simulink library "lib6DOFUtilityEquations"  (R2020b)
settings: Solver=VariableStepAuto  StartTime=0.0  StopTime=10.0  RelTol=1e-3
undefined symbols (not defined in the file): Earth, outputs, WGS84
libraries: aerolibtransform2 x1
settings Model: Creator=caatay  LastModifiedBy=caatay

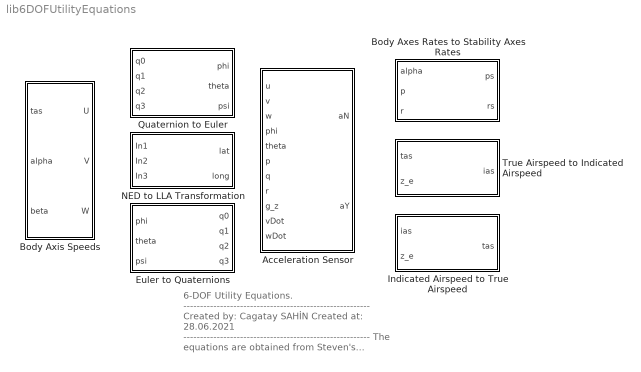
== system lib6DOFUtilityEquations ==
  note: 6-DOF Utility Equations.
      | --------------------------------------------------------
      | Created by: Cagatay SAHİN
      | Created at: 28.06.2021
      | --------------------------------------------------------
      | The equations are obtained from
      | Steven's textbook.
      | The reference book can be found in
      | "references folder".
      | --------------------------------------------------------
      | for question:
      | cagataysahin44@gmail.com
  Acceleration Sensor : Subsystem  mask(EOM Models - Utility Equations - Acceleration Sensor){}
      mask help: This block calculates acceleration information in SI Units.
      mask Help:
      | This block can calculate aircaft's acceleration data with using force and weight information
      | -------------------------------------------------------------------------------------------------------------------------------------------------
      | Inputs of this block:
      | 	u: X-Axis body speed (ft/sec)
      | 	v: Y-Axis body speed (ft/sec)
      | 	w: Z-Axis body speed (ft/sec)
      | 	phi: Roll Angle (rad)
      | 	theta: Pitch Angle (rad)
      | 	p: Body axis roll rate (ft/sec^2)
      | 	q: Body axis pitch rate (ft/sec^2)
      | 	r: Body axis yaw rate (ft/sec^2)
      | 	g_z: Z-Axis gravitional force (ft/sec^2)
      | 	vDot: Derivative of Y-Axis Body Speed (ft/sec^2)
      | 	wDot : Derivative of Z-Axis Body Speed (ft/sec^2)
      | Outputs of this block:
      | 	Aircraft acceleration: Z and Y acceleration [ft/sec^2].
      | -------------------------------------------------------------------------------------------------------------------------------------------------
      | Equations that in this block can be found in Steven's textbook. This textbook is in "literature" subfolder.
      | for question: "cagataysahin44@gmail.com".
      mask Display:
      | port_label('input',1,'u','texmode','on');
      | port_label('input',2,'v','texmode','on');
      | port_label('input',3,'w','texmode','on');
      | port_label('input',4,'\phi','texmode','on');
      | port_label('input',5,'\theta','texmode','on');
      | port_label('input',6,'p','texmode','on');
      | port_label('input',7,'q','texmode','on');
      | port_label('input',8,'r','texmode','on');
      | port_label('input',9,'g_{z}','texmode','on');
      | port_label('input',10,'v_{der}','texmode','on');
      | port_label('input',11,'w_{der}','texmode','on');
      | 
      | port_label('output',1,'a_{N}','texmode','on');
      | port_label('output',2,'a_{Y}','texmode','on');
  Body Axes Rates to Stability Axes Rates : Subsystem  mask(EOM Model - Utility Equations - Body Axes Rates to Stability Axes Rates){}
      mask help: Aircraft's stability axes angular rates calculation with using body axes angular rates and wind parameters alpha.
      mask Help:
      | This block can calculate aircaft's stability axes angular rates with using state information
      | -------------------------------------------------------------------------------------------------------------------------------------------------
      | Inputs of this block:
      | 	alpha: Angle of attack (rad).
      | 	p: Body axis roll rate (rad/s).
      | 	r: Body axis yaw rate (rad/s):
      | Outputs of this block:
      | 	p_s: Stability axis roll rate (rad/s).
      | 	r_s: Stabiltiy axis yaw rate (rad/s).
      | -------------------------------------------------------------------------------------------------------------------------------------------------
      | Equations that in this block can be found in Steven's textbook. This textbook is in "literature" subfolder.
      | for question: "cagataysahin44@gmail.com".
      mask Display:
      | port_label('input',1,'\alpha','texmode','on');
      | port_label('input',2,'p','texmode','on');
      | port_label('input',3,'r','texmode','on');
      | 
      | port_label('output',1,'p_{s}','texmode','on');
      | port_label('output',2,'r_{s}','texmode','on');
  Body Axis Speeds : Subsystem  mask(EOM Model - Utility Equations - Wind Paramaters to Body Axis Speeds.){}
      mask help: To Convert aircaft's wind parameters to body axis speeds which is coordinate transfer.
      mask Help:
      | This block can calculate aircaft's body axis speed which transforming wind axis coordinate to body axis coordinate.
      | -------------------------------------------------------------------------------------------------------------------------------------------------
      | Inputs of this block:
      | 	Wind Axis Params: Tas, AoA, AoS [ft/sec, rad].
      | Outputs of this block:
      | 	Body Axis Speeds: U, V, W body axis speeds [ft/sec].
      | -------------------------------------------------------------------------------------------------------------------------------------------------
      | Equations that in this block can be found in Steven's textbook. This textbook is in "literature" subfolder.
      | for question: "cagataysahin44@gmail.com".
      mask Display:
      | port_label('input',1,'V_{tas}','texmode','on');
      | port_label('input',2,'\alpha','texmode','on');
      | port_label('input',3,'\beta','texmode','on');
      | 
      | port_label('output',1,'U','texmode','on');
      | port_label('output',2,'V','texmode','on');
      | port_label('output',3,'W','texmode','on');
  Euler to Quaternions : Subsystem  mask(EOM Model - Utility Equations - Euler Angle to Quaternion Angle Transformation){}
      mask help: This function converts euler angles to quaternion angles.
      mask Help:
      | This block can transform euler angles to quaternion angles.
      | -------------------------------------------------------------------------------------------------------------------------------------------------
      | Inputs of this block:
      | 	Euler angles [rad].
      | Outputs of this block:
      | 	Quaternion angles [rad].
      | -------------------------------------------------------------------------------------------------------------------------------------------------
      | Equations that in this block can be found in Steven's textbook. This textbook is in "literature" subfolder.
      | for question: "cagataysahin44@gmail.com".
      mask Display:
      | port_label('input',1,'\phi','texmode','on');
      | port_label('input',2,'\theta','texmode','on');
      | port_label('input',3,'\psi','texmode','on');
      | 
      | port_label('output',1,'q_{0}','texmode','on');
      | port_label('output',2,'q_{1}','texmode','on');
      | port_label('output',3,'q_{2}','texmode','on');
      | port_label('output',4,'q_{3}','texmode','on');
  Indicated Airspeed to True Airspeed : Subsystem  mask(EOM Models - Utility Equations - IAS to TAS Conversion){}
      mask help: Aircraft's Lo-Fi True Airspeed calculation with using altitude and indicated airspeed information.
      mask Help:
      | This block can calculate aircaft's true airspeed with using state information.
      | -------------------------------------------------------------------------------------------------------------------------------------------------
      | Inputs of this block:
      | 	V_ias: Indicated airspeed (ft/sec)
      | 	z_e: Altitude (ft)
      | Outputs of this block:
      | 	V_tas: True airspeed (ft/sec)
      | -------------------------------------------------------------------------------------------------------------------------------------------------
      | Equations that in this block can be found in Steven's textbook. This textbook is in "literature" subfolder.
      | for question: "cagataysahin44@gmail.com".
      mask Display:
      | port_label('input',1,'V_{ias}','texmode','on');
      | port_label('input',2,'z_{e}','texmode','on');
      | 
      | port_label('output',1,'V_{tas}','texmode','on');
  NED to LLA Transformation : Subsystem  mask(EOM Model - Utility Equations -  NED tol LLA Transformation Model){}
      mask help: This function converts ned position variables (x,y,z) into lla (latitude, longitude, altitude) parameters.
      mask Help:
      | This block can transform North,East,Down values to Lattitude and Longitude angles.
      | -------------------------------------------------------------------------------------------------------------------------------------------------
      | Inputs of this block:
      | 	ned: North, East, Down values (ft).
      | Outputs of this block:
      | 	LLA: Latitude, Longitude (deg).
      | -------------------------------------------------------------------------------------------------------------------------------------------------
      | Equations that in this block can be found in Steven's textbook. This textbook is in "literature" subfolder.
      | for question: "cagataysahin44@gmail.com".
      mask Display:
      | port_label('input',1,'x_{e}','texmode','on');
      | port_label('input',2,'y_{e}','texmode','on');
      | port_label('input',3,'e_{e}','texmode','on');
      | 
      | port_label('output',1,'\mu','texmode','on');
      | port_label('output',2,'l','texmode','on');
  Quaternion to Euler : Subsystem  mask(EOM Model - Utility Equations -  Quaternion Angle to Euler Angle Transformation){}
      mask help: This function converts quaternion angles to euler angles.
      mask Help:
      | This block can transform quaternion angles to euler angles.
      | -------------------------------------------------------------------------------------------------------------------------------------------------
      | Inputs of this block:
      | 	Quaternion angles [rad].
      | Outputs of this block:
      | 	Euler angles [rad].
      | -------------------------------------------------------------------------------------------------------------------------------------------------
      | Equations that in this block can be found in Steven's textbook. This textbook is in "literature" subfolder.
      | for question: "cagataysahin44@gmail.com".
      mask Display:
      | port_label('output',1,'\phi','texmode','on');
      | port_label('output',2,'\theta','texmode','on');
      | port_label('output',3,'\psi','texmode','on');
      | 
      | port_label('input',1,'q_{0}','texmode','on');
      | port_label('input',2,'q_{1}','texmode','on');
      | port_label('input',3,'q_{2}','texmode','on');
      | port_label('input',4,'q_{3}','texmode','on');
  True Airspeed to Indicated Airspeed : Subsystem  mask(EOM Models - Utility Equations - TAS to IAS Conversion){}
      mask help: Aircraft's Lo-Fi Indicated Airspeed calculation with using altitude and true airspeed information.
      mask Help:
      | This block can calculate aircaft's indicated airspeed with using state information.
      | -------------------------------------------------------------------------------------------------------------------------------------------------
      | Inputs of this block:
      | 	V_tas: True airspeed (ft/sec)
      | 	z_e: Altitude (ft)
      | Outputs of this block:
      | 	V_ias: Indicated airspeed (ft/sec)
      | -------------------------------------------------------------------------------------------------------------------------------------------------
      | Equations that in this block can be found in Steven's textbook. This textbook is in "literature" subfolder.
      | for question: "cagataysahin44@gmail.com".
      mask Display:
      | port_label('input',1,'V_{tas}','texmode','on');
      | port_label('input',2,'z_{e}','texmode','on');
      | 
      | port_label('output',1,'V_{ias}','texmode','on');

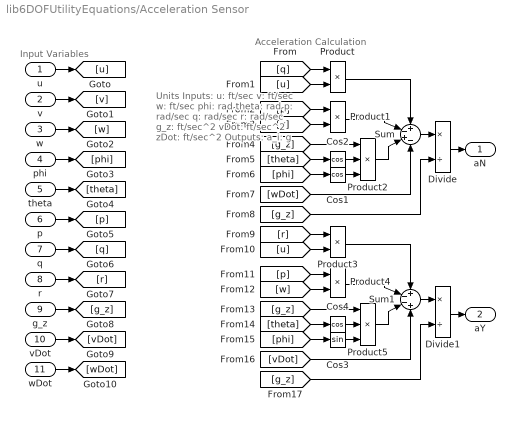
== system lib6DOFUtilityEquations/Acceleration Sensor ==
  note: Acceleration Calculation
  note: Input Variables
  note: Units
      | Inputs:
      | u: ft/sec
      | v: ft/sec
      | w: ft/sec
      | phi: rad
      | theta: rad
      | p: rad/sec
      | q: rad/sec
      | r: rad/sec
      | g_z: ft/sec^2
      | vDot: ft/sec^2
      | zDot: ft/sec^2
      | Outputs:
      | a_i: g
  u : Inport
  v : Inport  Port=2
  w : Inport  Port=3
  phi : Inport  Port=4
  theta : Inport  Port=5
  p : Inport  Port=6
  q : Inport  Port=7
  r : Inport  Port=8
  g_z : Inport  Port=9
  vDot : Inport  Port=10
  wDot : Inport  Port=11
  Cos1 : Trigonometry  Operator=cos
  Cos2 : Trigonometry  Operator=cos
  Cos3 : Trigonometry
  Cos4 : Trigonometry  Operator=cos
  Divide : Product  Inputs=*/
  Divide1 : Product  Inputs=*/
  Product{,1,3..4} (4 alike) : Product
  Product2 : Product  Inputs=3
  Product5 : Product  Inputs=3
  Sum : Sum  Inputs=+-+-
  Sum1 : Sum  Inputs=+--+
  aN : Outport
  aY : Outport  Port=2
  wires:
  u/1 -> [u]
  v/1 -> [v]
  theta/1 -> [theta]
  phi/1 -> [phi]
  w/1 -> [w]
  p/1 -> [p]
  q/1 -> [q]
  r/1 -> [r]
  wDot/1 -> [wDot]
  vDot/1 -> [vDot]
  g_z/1 -> [g_z]
  [q] -> Product/1
  [u] -> Product/2
  [p] -> Product1/1
  [v] -> Product1/2
  [theta] -> Cos2/1
  [phi] -> Cos1/1
  [g_z] -> Product2/1
  Cos2/1 -> Product2/2
  Cos1/1 -> Product2/3
  [wDot] -> Sum/4
  Product1/1 -> Sum/2
  Product/1 -> Sum/1
  Product2/1 -> Sum/3
  [g_z] -> Divide/2
  Sum/1 -> Divide/1
  Divide/1 -> aN/1
  [w] -> Product4/2
  Divide1/1 -> aY/1
  Cos4/1 -> Product5/2
  Cos3/1 -> Product5/3
  Sum1/1 -> Divide1/1
  [phi] -> Cos3/1
  Product4/1 -> Sum1/2
  [r] -> Product3/1
  Product5/1 -> Sum1/3
  [u] -> Product3/2
  [g_z] -> Product5/1
  [vDot] -> Sum1/4
  Product3/1 -> Sum1/1
  [p] -> Product4/1
  [g_z] -> Divide1/2
  [theta] -> Cos4/1

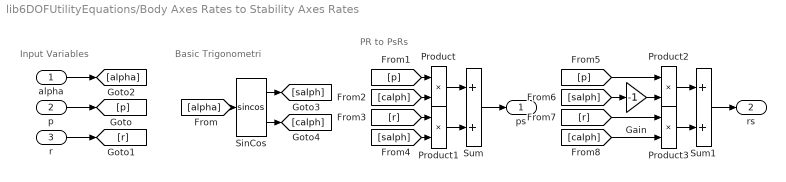
== system lib6DOFUtilityEquations/Body Axes Rates to Stability Axes Rates ==
  note: Basic Trigonometri
  note: Input Variables
  note: PR to PsRs
  alpha : Inport
  p : Inport  Port=2
  r : Inport  Port=3
  Gain : Gain  Gain=-1
  Product{,1..3} (4 alike) : Product
  SinCos : Trigonometry  Operator=sincos
  Sum : Sum
  Sum1 : Sum
  ps : Outport
  rs : Outport  Port=2
  wires:
  r/1 -> [r]
  p/1 -> [p]
  alpha/1 -> [alpha]
  [alpha] -> SinCos/1
  SinCos/1 -> [salph]
  SinCos/2 -> [calph]
  [calph] -> Product/2
  [p] -> Product/1
  [r] -> Product1/1
  [salph] -> Product1/2
  Product1/1 -> Sum/2
  Product/1 -> Sum/1
  Sum/1 -> ps/1
  Product2/1 -> Sum1/1
  [calph] -> Product3/2
  [salph] -> Gain/1
  [p] -> Product2/1
  Product3/1 -> Sum1/2
  Sum1/1 -> rs/1
  [r] -> Product3/1
  Gain/1 -> Product2/2

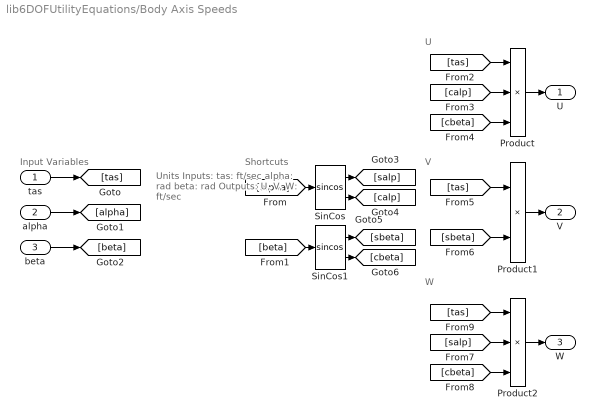
== system lib6DOFUtilityEquations/Body Axis Speeds ==
  note: V
  note: Shortcuts
  note: Input Variables
  note: Units
      | Inputs:
      | tas: ft/sec
      | alpha: rad
      | beta: rad
      | Outputs:
      | U, V, W: ft/sec
  note: U
  note: W
  "tas " : Inport
  alpha : Inport  Port=2
  beta : Inport  Port=3
  Product : Product  Inputs=3
  Product1 : Product
  Product2 : Product  Inputs=3
  SinCos : Trigonometry  Operator=sincos
  SinCos1 : Trigonometry  Operator=sincos
  U : Outport  VectorParamsAs1DForOutWhenUnconnected=off
  V : Outport  Port=2  VectorParamsAs1DForOutWhenUnconnected=off
  W : Outport  Port=3  VectorParamsAs1DForOutWhenUnconnected=off
  wires:
  alpha/1 -> [alpha]
  beta/1 -> [beta]
  "tas "/1 -> [tas]
  [alpha] -> SinCos/1
  [beta] -> SinCos1/1
  SinCos/1 -> [salp]
  SinCos/2 -> [calp]
  SinCos1/1 -> [sbeta]
  SinCos1/2 -> [cbeta]
  [cbeta] -> Product/3
  [calp] -> Product/2
  [tas] -> Product/1
  Product/1 -> U/1
  [tas] -> Product1/1
  [sbeta] -> Product1/2
  Product1/1 -> V/1
  Product2/1 -> W/1
  [salp] -> Product2/2
  [cbeta] -> Product2/3
  [tas] -> Product2/1

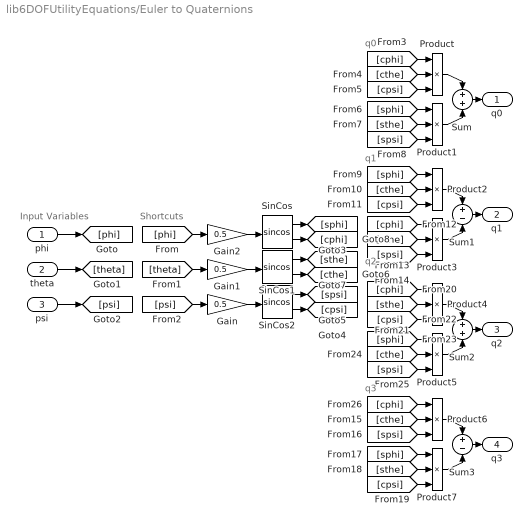
== system lib6DOFUtilityEquations/Euler to Quaternions ==
  note: q0
  note: Shortcuts
  note: Input Variables
  note: q1
  note: q3
  note: q2
  phi : Inport
  theta : Inport  Port=2
  psi : Inport  Port=3
  Gain : Gain  Gain=0.5
  Gain1 : Gain  Gain=0.5
  Gain2 : Gain  Gain=0.5
  Product{,1..7} (8 alike) : Product  Inputs=3
  SinCos : Trigonometry  Operator=sincos
  SinCos1 : Trigonometry  Operator=sincos
  SinCos2 : Trigonometry  Operator=sincos
  Sum : Sum
  Sum1 : Sum  Inputs=+-
  Sum2 : Sum
  Sum3 : Sum  Inputs=+-
  q0 : Outport  VectorParamsAs1DForOutWhenUnconnected=off
  q1 : Outport  Port=2  VectorParamsAs1DForOutWhenUnconnected=off
  q2 : Outport  Port=3  VectorParamsAs1DForOutWhenUnconnected=off
  q3 : Outport  Port=4  VectorParamsAs1DForOutWhenUnconnected=off
  wires:
  phi/1 -> [phi]
  theta/1 -> [theta]
  psi/1 -> [psi]
  [psi] -> Gain/1
  [theta] -> Gain1/1
  [phi] -> Gain2/1
  Gain2/1 -> SinCos/1
  Gain1/1 -> SinCos1/1
  Gain/1 -> SinCos2/1
  SinCos/1 -> [sphi]
  SinCos2/2 -> [cpsi]
  SinCos2/1 -> [spsi]
  SinCos1/2 -> [cthe]
  SinCos1/1 -> [sthe]
  SinCos/2 -> [cphi]
  [cphi] -> Product/1
  [cthe] -> Product/2
  [cpsi] -> Product/3
  [sthe] -> Product1/2
  [spsi] -> Product1/3
  [sphi] -> Product1/1
  Product1/1 -> Sum/2
  Product/1 -> Sum/1
  Sum/1 -> q0/1
  Sum1/1 -> q1/1
  [cthe] -> Product2/2
  [sphi] -> Product2/1
  Product2/1 -> Sum1/1
  [sthe] -> Product3/2
  Product3/1 -> Sum1/2
  [cphi] -> Product3/1
  [cpsi] -> Product2/3
  Product5/1 -> Sum2/2
  Product6/1 -> Sum3/1
  [sphi] -> Product7/1
  [spsi] -> Product6/3
  Product7/1 -> Sum3/2
  [cphi] -> Product6/1
  Sum3/1 -> q3/1
  [sthe] -> Product4/2
  [cphi] -> Product4/1
  Product4/1 -> Sum2/1
  [cthe] -> Product5/2
  [spsi] -> Product5/3
  [sthe] -> Product7/2
  Sum2/1 -> q2/1
  [cthe] -> Product6/2
  [sphi] -> Product5/1
  [cpsi] -> Product4/3
  [cpsi] -> Product7/3
  [spsi] -> Product3/3

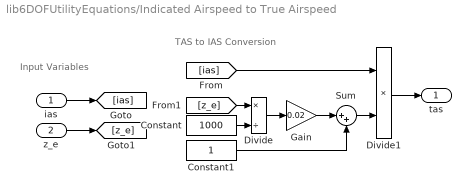
== system lib6DOFUtilityEquations/Indicated Airspeed to True Airspeed ==
  note: TAS to IAS Conversion
  note: Input Variables
  ias : Inport
  z_e : Inport  Port=2
  Constant : Constant  Value=1000
  Constant1 : Constant
  Divide : Product  Inputs=*/
  Divide1 : Product  Inputs=**
  Gain : Gain  Gain=0.02
  Sum : Sum  Inputs=|++
  tas : Outport
  wires:
  z_e/1 -> [z_e]
  ias/1 -> [ias]
  Divide1/1 -> tas/1
  [z_e] -> Divide/1
  Constant/1 -> Divide/2
  Divide/1 -> Gain/1
  Gain/1 -> Sum/1
  Sum/1 -> Divide1/2
  Constant1/1 -> Sum/2
  [ias] -> Divide1/1

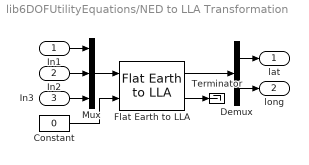
== system lib6DOFUtilityEquations/NED to LLA Transformation ==
  In1 : Inport
  In2 : Inport  Port=2
  In3 : Inport  Port=3
  Constant : Constant  Value=0
  Demux : Demux  Outputs=2
  Flat Earth to LLA : aerolibtransform2/Flat Earth to LLA  units=Metric (MKS)  ptype=Earth (WGS84)  F=1/298.257223563  R=6378137  refPosPort=off  LL0=[outputs.trim.states.lat outputs.trim.states.long]  psi=0
  Mux : Mux  Inputs=3
  Terminator : Terminator
  lat : Outport
  long : Outport  Port=2
  wires:
  In2/1 -> Mux/2
  In1/1 -> Mux/1
  In3/1 -> Mux/3
  Mux/1 -> Flat Earth to LLA/1
  Constant/1 -> Flat Earth to LLA/2
  Flat Earth to LLA/2 -> Terminator/1
  Flat Earth to LLA/1 -> Demux/1
  Demux/1 -> lat/1
  Demux/2 -> long/1

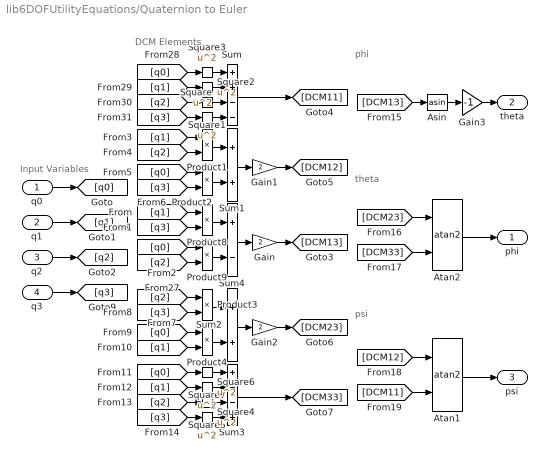
== system lib6DOFUtilityEquations/Quaternion to Euler ==
  note: phi
  note: DCM Elements
  note: Input Variables
  note: theta
  note: psi
  q0 : Inport
  q1 : Inport  Port=2
  q2 : Inport  Port=3
  q3 : Inport  Port=4
  Asin : Trigonometry  Operator=asin
  Atan1 : Trigonometry  Operator=atan2
  Atan2 : Trigonometry  Operator=atan2
  Gain : Gain  Gain=2
  Gain1 : Gain  Gain=2
  Gain2 : Gain  Gain=2
  Gain3 : Gain  Gain=-1
  Product{1..4,8..9} (6 alike) : Product
  Square{,1..7} (8 alike) : Math  Operator=square  SignedPower=on  SaturateOnIntegerOverflow=on
  Sum : Sum  Inputs=++--
  Sum1 : Sum
  Sum2 : Sum
  Sum3 : Sum  Inputs=+--+
  Sum4 : Sum  Inputs=+-
  phi : Outport  VectorParamsAs1DForOutWhenUnconnected=off
  theta : Outport  Port=2  VectorParamsAs1DForOutWhenUnconnected=off
  psi : Outport  Port=3  VectorParamsAs1DForOutWhenUnconnected=off
  wires:
  q1/1 -> [q1]
  q2/1 -> [q2]
  q0/1 -> [q0]
  q3/1 -> [q3]
  [q1] -> Product8/1
  [q2] -> Product9/2
  [q0] -> Product9/1
  [q3] -> Product8/2
  Product9/1 -> Sum4/2
  Product8/1 -> Sum4/1
  Sum4/1 -> Gain/1
  Gain/1 -> [DCM13]
  [q2] -> Square1/1
  Sum/1 -> [DCM11]
  [q3] -> Square/1
  [q0] -> Square3/1
  [q1] -> Square2/1
  Square/1 -> Sum/4
  Square1/1 -> Sum/3
  Square2/1 -> Sum/2
  Square3/1 -> Sum/1
  [q0] -> Product2/1
  Sum1/1 -> Gain1/1
  Gain1/1 -> [DCM12]
  Product2/1 -> Sum1/2
  [q3] -> Product2/2
  Product1/1 -> Sum1/1
  [q1] -> Product1/1
  [q2] -> Product1/2
  [q0] -> Product4/1
  Sum2/1 -> Gain2/1
  Gain2/1 -> [DCM23]
  Product4/1 -> Sum2/2
  [q1] -> Product4/2
  Product3/1 -> Sum2/1
  [q2] -> Product3/1
  [q3] -> Product3/2
  [q3] -> Square4/1
  Square6/1 -> Sum3/2
  [q1] -> Square6/1
  Sum3/1 -> [DCM33]
  Square5/1 -> Sum3/3
  Square4/1 -> Sum3/4
  [q2] -> Square5/1
  [q0] -> Square7/1
  Square7/1 -> Sum3/1
  Asin/1 -> Gain3/1
  Gain3/1 -> theta/1
  Atan1/1 -> psi/1
  Atan2/1 -> phi/1
  [DCM13] -> Asin/1
  [DCM23] -> Atan2/1
  [DCM33] -> Atan2/2
  [DCM12] -> Atan1/1
  [DCM11] -> Atan1/2

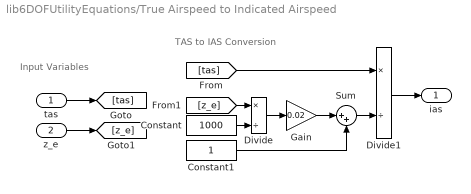
== system lib6DOFUtilityEquations/True Airspeed to Indicated Airspeed ==
  note: TAS to IAS Conversion
  note: Input Variables
  tas : Inport
  z_e : Inport  Port=2
  Constant : Constant  Value=1000
  Constant1 : Constant
  Divide : Product  Inputs=*/
  Divide1 : Product  Inputs=*/
  Gain : Gain  Gain=0.02
  Sum : Sum  Inputs=|++
  ias : Outport
  wires:
  tas/1 -> [tas]
  z_e/1 -> [z_e]
  Constant/1 -> Divide/2
  [z_e] -> Divide/1
  Divide/1 -> Gain/1
  Gain/1 -> Sum/1
  Constant1/1 -> Sum/2
  Sum/1 -> Divide1/2
  [tas] -> Divide1/1
  Divide1/1 -> ias/1
